simulink model "V1"  (R2025a)
settings: Solver=VariableStepAuto  StartTime=0.0  StopTime=200  FixedStep=0.005  RelTol=1e-3
libraries: cstblocks x11, vrlib x10, slpidlib x9, simulink_extras x8, dspinverses x3, robotcorelib x2, simulink x1
(part 3 of 3)

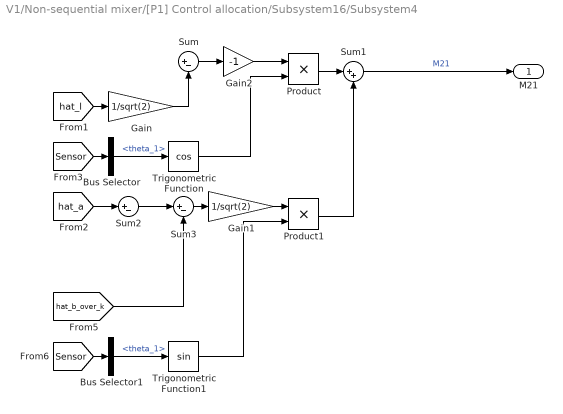
== system V1/Non-sequential mixer/[P1] Control allocation/Subsystem16/Subsystem4 ==
  Bus Selector : BusSelector  OutputSignals=theta_1
  Bus Selector1 : BusSelector  OutputSignals=theta_1
  Gain : Gain  Gain=1/sqrt(2)
  Gain1 : Gain  Gain=1/sqrt(2)
  Gain2 : Gain  Gain=-1
  Product : Product
  Product1 : Product
  Sum : Sum  Inputs=|+-
  Sum1 : Sum  Inputs=|++
  Sum2 : Sum  Inputs=|+-
  Sum3 : Sum  Inputs=|+-
  Trigonometric Function : Trigonometry  Operator=cos
  Trigonometric Function1 : Trigonometry
  M21 : Outport
  wires:
  Product/1 -> Sum1/1
  Sum/1 -> Gain2/1
  Sum2/1 -> Sum3/1
  Trigonometric Function/1 -> Product/2
  Bus Selector/1 -> Trigonometric Function/1  "<theta_1>"
  [hat_a] -> Sum2/1
  Gain/1 -> Sum/2
  Sum3/1 -> Gain1/1
  [hat_b_over_k] -> Sum3/2
  Gain1/1 -> Product1/1
  [hat_l] -> Gain/1
  Product1/1 -> Sum1/2
  Trigonometric Function1/1 -> Product1/2
  Bus Selector1/1 -> Trigonometric Function1/1  "<theta_1>"
  [Sensor] -> Bus Selector/1
  [Sensor] -> Bus Selector1/1
  Sum1/1 -> M21/1  "M21"
  Gain2/1 -> Product/1

== system V1/Non-sequential mixer/[P1] Control allocation/Subsystem16/Subsystem5 ==
  Bus Selector : BusSelector  OutputSignals=theta_2
  Bus Selector1 : BusSelector  OutputSignals=theta_2
  Gain : Gain  Gain=1/sqrt(2)
  Gain1 : Gain  Gain=1/sqrt(2)
  Gain2 : Gain  Gain=-1
  Product : Product
  Product1 : Product
  Sum : Sum  Inputs=|++
  Sum1 : Sum  Inputs=|++
  Sum2 : Sum  Inputs=|+-
  Sum3 : Sum  Inputs=|+-
  Trigonometric Function : Trigonometry  Operator=cos
  Trigonometric Function1 : Trigonometry
  M22 : Outport
  wires:
  Product/1 -> Sum1/1
  Sum/1 -> Gain2/1
  Sum2/1 -> Sum3/1
  Trigonometric Function/1 -> Product/2
  Bus Selector/1 -> Trigonometric Function/1  "<theta_2>"
  [hat_a] -> Sum2/1
  Gain/1 -> Sum/2
  Sum3/1 -> Gain1/1
  [hat_b_over_k] -> Sum3/2
  Gain1/1 -> Product1/1
  [hat_l] -> Gain/1
  Product1/1 -> Sum1/2
  Trigonometric Function1/1 -> Product1/2
  Bus Selector1/1 -> Trigonometric Function1/1  "<theta_2>"
  [Sensor] -> Bus Selector/1
  [Sensor] -> Bus Selector1/1
  Sum1/1 -> M22/1  "M22"
  Gain2/1 -> Product/1

== system V1/Non-sequential mixer/[P1] Control allocation/Subsystem16/Subsystem6 ==
  Bus Selector : BusSelector  OutputSignals=theta_3
  Bus Selector1 : BusSelector  OutputSignals=theta_3
  Gain : Gain  Gain=1/sqrt(2)
  Gain1 : Gain  Gain=1/sqrt(2)
  Gain2 : Gain  Gain=-1
  Product : Product
  Product1 : Product
  Sum : Sum  Inputs=|++
  Sum1 : Sum  Inputs=|++
  Sum2 : Sum  Inputs=|+-
  Sum3 : Sum  Inputs=|-+
  Trigonometric Function : Trigonometry  Operator=cos
  Trigonometric Function1 : Trigonometry
  M23 : Outport
  wires:
  Product/1 -> Sum1/1
  Sum/1 -> Gain2/1
  Sum2/1 -> Sum3/1
  Trigonometric Function/1 -> Product/2
  Bus Selector/1 -> Trigonometric Function/1  "<theta_3>"
  [hat_a] -> Sum2/1
  Gain/1 -> Sum/2
  Sum3/1 -> Gain1/1
  [hat_b_over_k] -> Sum3/2
  Gain1/1 -> Product1/1
  [hat_l] -> Gain/1
  Product1/1 -> Sum1/2
  Trigonometric Function1/1 -> Product1/2
  Bus Selector1/1 -> Trigonometric Function1/1  "<theta_3>"
  [Sensor] -> Bus Selector/1
  [Sensor] -> Bus Selector1/1
  Sum1/1 -> M23/1  "M23"
  Gain2/1 -> Product/1

== system V1/Non-sequential mixer/[P1] Control allocation/Subsystem16/Subsystem7 ==
  Bus Selector : BusSelector  OutputSignals=theta_4
  Bus Selector1 : BusSelector  OutputSignals=theta_4
  Gain : Gain  Gain=1/sqrt(2)
  Gain1 : Gain  Gain=1/sqrt(2)
  Gain2 : Gain  Gain=-1
  Product : Product
  Product1 : Product
  Sum : Sum  Inputs=|+-
  Sum1 : Sum  Inputs=|++
  Sum2 : Sum  Inputs=|+-
  Sum3 : Sum  Inputs=|-+
  Trigonometric Function : Trigonometry  Operator=cos
  Trigonometric Function1 : Trigonometry
  M24 : Outport
  wires:
  Product/1 -> Sum1/1
  Sum/1 -> Gain2/1
  Sum2/1 -> Sum3/1
  Trigonometric Function/1 -> Product/2
  Bus Selector/1 -> Trigonometric Function/1  "<theta_4>"
  [hat_a] -> Sum2/1
  Gain/1 -> Sum/2
  Sum3/1 -> Gain1/1
  [hat_b_over_k] -> Sum3/2
  Gain1/1 -> Product1/1
  [hat_l] -> Gain/1
  Product1/1 -> Sum1/2
  Trigonometric Function1/1 -> Product1/2
  Bus Selector1/1 -> Trigonometric Function1/1  "<theta_4>"
  [Sensor] -> Bus Selector/1
  [Sensor] -> Bus Selector1/1
  Sum1/1 -> M24/1  "M24"
  Gain2/1 -> Product/1

== system V1/Non-sequential mixer/[P1] Control allocation/Subsystem16/Subsystem8 ==
  Bus Selector : BusSelector  OutputSignals=theta_1
  Product2 : Product
  Trigonometric Function : Trigonometry  Operator=cos
  M31 : Outport
  wires:
  Bus Selector/1 -> Trigonometric Function/1  "<theta_1>"
  [Sensor] -> Bus Selector/1
  Trigonometric Function/1 -> Product2/2
  [hat_b_over_k] -> Product2/1
  Product2/1 -> M31/1

== system V1/Non-sequential mixer/[P1] Control allocation/Subsystem16/Subsystem9 ==
  Bus Selector : BusSelector  OutputSignals=theta_2
  Gain : Gain  Gain=-1
  Product2 : Product
  Trigonometric Function : Trigonometry  Operator=cos
  M32 : Outport
  wires:
  Bus Selector/1 -> Trigonometric Function/1  "<theta_2>"
  [Sensor] -> Bus Selector/1
  Trigonometric Function/1 -> Product2/2
  [hat_b_over_k] -> Product2/1
  Product2/1 -> Gain/1
  Gain/1 -> M32/1
